simulink model "Levitazione_Elettromagnetica_retroazione"  (Simulink 7.1)
settings: Solver=ode45  StartTime=0.0  StopTime=10.0  MaxStep=1e-4  RelTol=1e-3
values from neighbouring files (symbols this model uses):
  A = N    (= 20)    [Dati_Levitazione.m]    (also in Dati_Levitazione_retroazione.m)
  B = 2*H0_E    [Dati_Levitazione.m]    (also in Dati_Levitazione_retroazione.m)
  C = (Lf+2*x_E*(MU_D/MU_0))*(M/(2*S*MU_D*H0_E))    [Dati_Levitazione.m]    (also in Dati_Levitazione_retroazione.m)
  Kd = C*(s1+s2+s3)/A    [Dati_Levitazione_retroazione.m]
  Ki = (C*s1*s2*s3)/A    [Dati_Levitazione_retroazione.m]
  Kp = -(B+C*(s1*s2+s2*s3+s3*s1))/A    [Dati_Levitazione_retroazione.m]
libraries: simulink x2
settings Model: Creator=elettrica  LastModifiedBy=elettrica

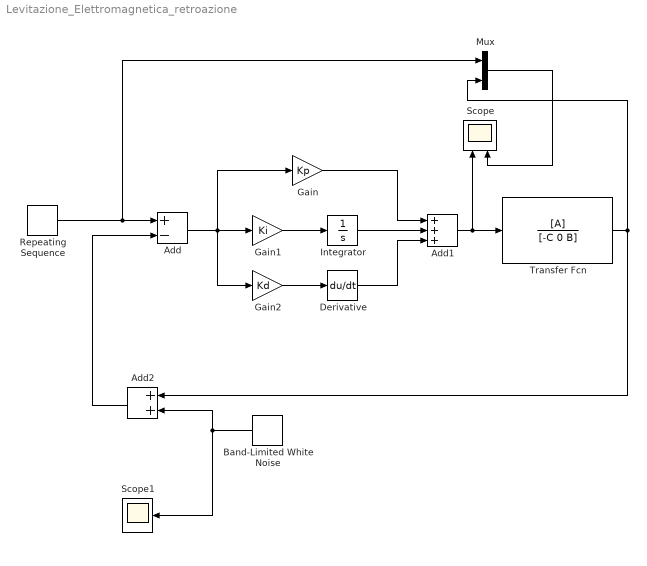
== system Levitazione_Elettromagnetica_retroazione ==
  Add : Sum  Inputs=+-  OutDataType=sfix(16)  OutScaling=2^-10
  Add1 : Sum  Inputs=+++  OutDataType=sfix(16)  OutScaling=2^-10
  Add2 : Sum  Orientation=left  OutDataType=sfix(16)  OutScaling=2^-10
  Band-Limited White Noise : simulink/Sources/Band-Limited White Noise  Orientation=left  SystemSampleTime=-1  Cov=[0.000000001]  Ts=0.01  seed=[14311]
  Derivative : Derivative
  Gain : Gain  Gain=Kp  ParameterDataType=sfix(16)  ParameterScaling=2^0  OutDataType=sfix(16)  OutScaling=2^0
  Gain1 : Gain  Gain=Ki  ParameterDataType=sfix(16)  ParameterScaling=2^0  OutDataType=sfix(16)  OutScaling=2^0
  Gain2 : Gain  Gain=Kd  ParameterDataType=sfix(16)  ParameterScaling=2^0  OutDataType=sfix(16)  OutScaling=2^0
  Integrator : Integrator
  Mux : Mux  Inputs=2
  Repeating Sequence : simulink/Sources/Repeating Sequence  SystemSampleTime=-1  rep_seq_t=[0 1 2 3 4]  rep_seq_y=[0 0 -0.005 -0.005 0]
  Scope : Scope  NumInputPorts=2
      settings: Orientation=up  YMin=-5~-5  YMax=5~5
  Scope1 : Scope
  Transfer Fcn : TransferFcn  Numerator=[A]  Denominator=[-C 0 B]
  wires:
  Transfer Fcn/1 -> Mux/2, Add2/1
  Repeating Sequence/1 -> Add/1, Mux/1
  Gain/1 -> Add1/1
  Integrator/1 -> Add1/2
  Derivative/1 -> Add1/3
  Add1/1 -> Transfer Fcn/1, Scope/1
  Gain1/1 -> Integrator/1
  Gain2/1 -> Derivative/1
  Add/1 -> Gain1/1, Gain2/1, Gain/1
  Mux/1 -> Scope/2
  Band-Limited White Noise/1 -> Add2/2, Scope1/1
  Add2/1 -> Add/2
